simulink model "digital9"  (R2024a)
settings: Solver=VariableStepAuto  StartTime=0.0  StopTime=10.0  RelTol=1e-3
settings Model: Creator=tusha  LastModifiedBy=tusha

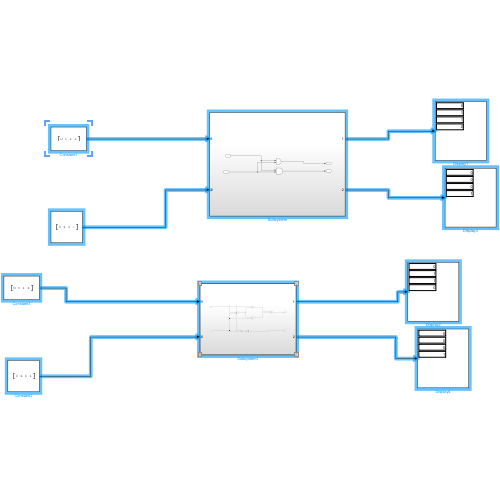
[thumbnail: Simulink's stored preview of the top-level diagram]
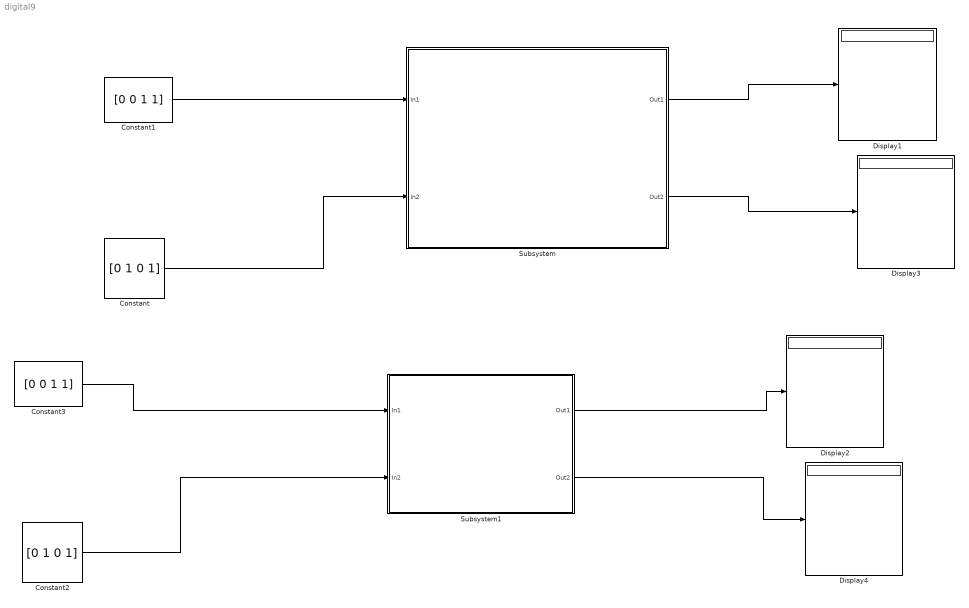
== system digital9 ==
  Constant : Constant  Value=[0 1 0 1]
  Constant1 : Constant  Value=[0 0 1 1]
  Constant2 : Constant  Value=[0 1 0 1]
  Constant3 : Constant  Value=[0 0 1 1]
  Display{1..4} (4 alike) : Display
  Subsystem : Subsystem
  Subsystem1 : Subsystem
  wires:
  Constant1/1 -> Subsystem/1(In1)
  Constant/1 -> Subsystem/2(In2)
  Subsystem/2(Out2) -> Display3/1
  Subsystem/1(Out1) -> Display1/1
  Constant3/1 -> Subsystem1/1(In1)
  Constant2/1 -> Subsystem1/2(In2)
  Subsystem1/1(Out1) -> Display2/1
  Subsystem1/2(Out2) -> Display4/1

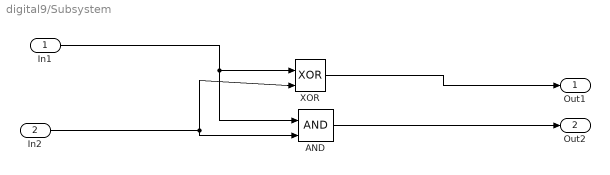
== system digital9/Subsystem ==
  In1 : Inport
  In2 : Inport  Port=2
  AND : Logic  IconShape=distinctive  AllPortsSameDT=off  OutDataTypeStr=boolean
  XOR : Logic  Operator=XOR  IconShape=distinctive  AllPortsSameDT=off  OutDataTypeStr=boolean
  Out1 : Outport
  Out2 : Outport  Port=2
  wires:
  In1/1 -> AND/1, XOR/1
  In2/1 -> XOR/2, AND/2
  AND/1 -> Out2/1
  XOR/1 -> Out1/1

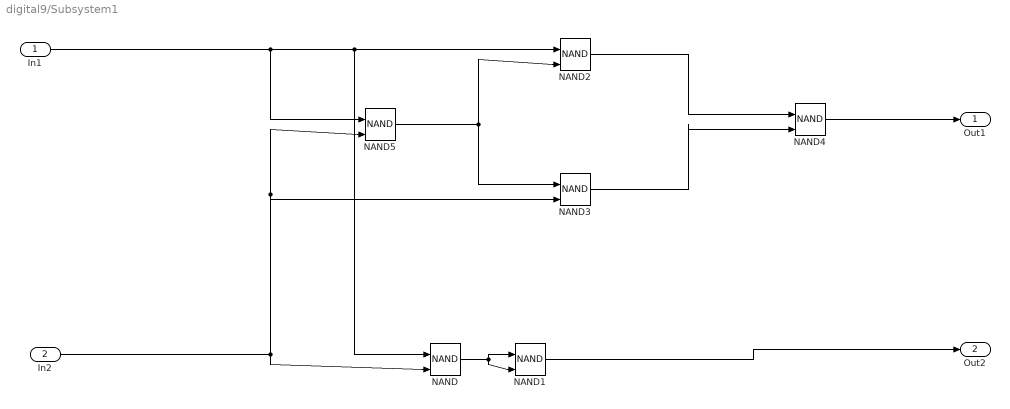
== system digital9/Subsystem1 ==
  In1 : Inport
  In2 : Inport  Port=2
  NAND{,1..5} (6 alike) : Logic  Operator=NAND  IconShape=distinctive  AllPortsSameDT=off  OutDataTypeStr=boolean
  Out1 : Outport
  Out2 : Outport  Port=2
  wires:
  In2/1 -> NAND5/2, NAND3/2, NAND/2
  NAND/1 -> NAND1/1, NAND1/2
  NAND1/1 -> Out2/1
  NAND2/1 -> NAND4/1
  NAND3/1 -> NAND4/2
  NAND5/1 -> NAND2/2, NAND3/1
  In1/1 -> NAND/1, NAND2/1, NAND5/1
  NAND4/1 -> Out1/1
